simulink model "compSR"  (Simulink 6.4)
settings: Solver=ode4  StartTime=0.0  StopTime=cas_simulacie  FixedStep=ptv_sim_step  RelTol=1e-3
values from neighbouring files (symbols this model uses):
  D = D_km    [id_model3.m]    (also in id_tune.m = 0.1; id_tune_pe_zal.m = id_backup(4))
  K = get(findobj('Tag','ptt_s4'),'Value')    [id_tune.m]    (also in id_tune_pe_zal.m = id_backup(2); id_tune_zal.m = y_norm(end); km_id.m = 0; km_sustavy.m = y_nek)
  M = (y_max-y_min)/y_max    [km_id.m]    (also in km_sustavy.m)
settings Model: Creator=oravec  LastModifiedBy=oravec
settings DataIOCC: LimitDataPoints=off  SignalLoggingName=sigsOut
settings OptimizationCC: InitFltsAndDblsToZero=off
settings DebuggingCC: SolverPrmCheckMsg=none  StrictBusMsg=None
settings HardwareCC: TargetHWDeviceType=32-bit Generic  TargetUnknown=on  ProdEqTarget=off

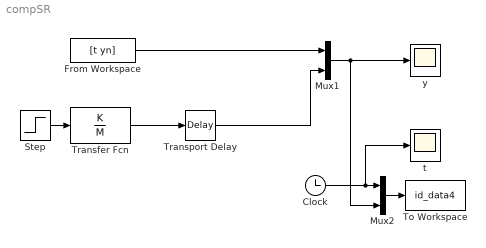
== system compSR ==
  Clock : Clock
      settings: Decimation=10
  From Workspace : FromWorkspace  VariableName=[t yn]  SampleTime=0
  Mux1 : Mux  Inputs=2
  Mux2 : Mux  Inputs=2
  Step : Step  Time=0  SampleTime=0
  To Workspace : ToWorkspace  VariableName=id_data4  SampleTime=-1  SaveFormat=Array
  Transfer Fcn : TransferFcn  Numerator=K  Denominator=M
  Transport Delay : TransportDelay  DelayTime=D
  t : Scope
  y : Scope
  wires:
  Transfer Fcn/1 -> Transport Delay/1
  Step/1 -> Transfer Fcn/1
  Mux1/1 -> y/1, Mux2/2
  Mux2/1 -> To Workspace/1
  Transport Delay/1 -> Mux1/2
  From Workspace/1 -> Mux1/1
  Clock/1 -> Mux2/1, t/1
